simulink model "WashMachine"  (R2020b)
settings: Solver=VariableStepAuto  StartTime=0.0  StopTime=10.0  RelTol=1e-3
settings Model: EnablePacing=on  PacingRate=0.500000  Creator=apple  LastModifiedBy=apple

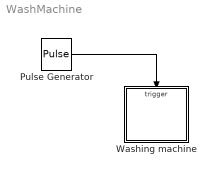
== system WashMachine ==
  Pulse Generator : DiscretePulseGenerator  PulseType=Time based  Amplitude=[1,1,1]  Period=[10,10,10]  PulseWidth=[5,5,5]  PhaseDelay=[0,0,0]
  Washing machine : Stateflow chart  TreatAsAtomicUnit=on
  wires:
  Pulse Generator/1 -> Washing machine/Trigger

== stateflow chart WashMachine/Washing machine ==
  settings: executeAtInitialization=1
  state OFF
    state Ready
      en:fprintf("Initialization");n3 = 45;
    state off
      en:time = 0;
      finish = 0;
    state Pending_State
      en:fprintf("pending")
    (default) -> off
    off -> Ready : START
    Pending_State -> off [order 2] : STOP
  state ON
    on E:fprintf("Washing Completed!");
    (history)
    state Add_Water
      du:time = time + 1;
      en:fprintf("Entry stage1")
    state Washing
      du:time = time + 1;
      en:fprintf("Entry stage2")
    Add_Water -> Washing : [time >= 5]/{time = 0;}
    Washing -> Add_Water : [time >= 10]/{time = 0;}
  (default) -> OFF
  Ready -> Add_Water : SWITCH
  ON -> OFF [order 1] : STOP
  ON -> OFF [order 3] : after(n3,sec)[finish == 0]{finish = 1;send(E);}
  Pending_State -> ON [order 1] : SWITCH
  ON -> Pending_State [order 2] : SWITCH{n3 = n3 - temporalCount(sec)}
  data: n1 local =5; n2 local =10; n3 local =45; finish local; time local
  events: E local FUNCTION_CALL_EVENT; SWITCH input EITHER_EDGE_EVENT; START input EITHER_EDGE_EVENT; STOP input EITHER_EDGE_EVENT
